simulink subsystem "Accelerometer_SubSystem"  (R2020b)
settings: Solver=VariableStepAuto  StartTime=0.0  StopTime=10.0  RelTol=1e-3
undefined symbols (not defined in the file): g, ms22g, sens, Ts, wheel
settings Model: Creator=umberto  LastModifiedBy=Musta

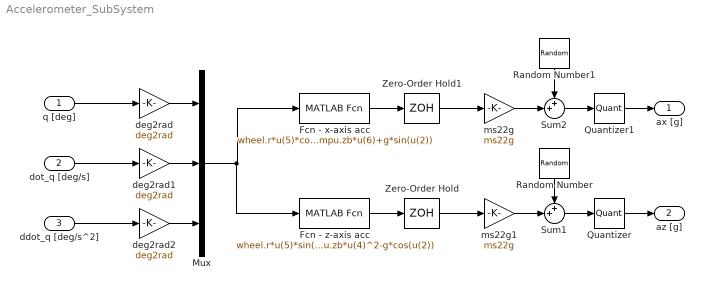
== system Accelerometer_SubSystem ==
  q [deg] : Inport
  dot_q [deg/s] : Inport  Port=2
  ddot_q [deg/s^2] : Inport  Port=3
  Fcn - x-axis acc : MATLABFcn  MATLABFcn=wheel.r*u(5)*cos(u(2))+sens.mpu.zb*u(6)+g*sin(u(2))
  Fcn - z-axis acc : MATLABFcn  MATLABFcn=wheel.r*u(5)*sin(u(2))-sens.mpu.zb*u(4)^2-g*cos(u(2))
  Mux : Mux  Inputs=3
  Quantizer : Quantizer  QuantizationInterval=sens.mpu.acc.LSB2g
  Quantizer1 : Quantizer  QuantizationInterval=sens.mpu.acc.LSB2g
  Random Number : RandomNumber  Variance=sens.mpu.acc.noisevar  SampleTime=Ts
  Random Number1 : RandomNumber  Variance=sens.mpu.acc.noisevar  SampleTime=Ts
  Sum1 : Sum  Inputs=++|
  Sum2 : Sum  Inputs=++|
  Zero-Order Hold : ZeroOrderHold  SampleTime=Ts
  Zero-Order Hold1 : ZeroOrderHold  SampleTime=Ts
  deg2rad : Gain  Gain=deg2rad
  deg2rad1 : Gain  Gain=deg2rad
  deg2rad2 : Gain  Gain=deg2rad
  ms22g : Gain  Gain=ms22g
  ms22g1 : Gain  Gain=ms22g
  ax [g] : Outport
  az [g] : Outport  Port=2
  wires:
  q [deg]/1 -> deg2rad/1
  dot_q [deg/s]/1 -> deg2rad1/1
  ddot_q [deg/s^2]/1 -> deg2rad2/1
  deg2rad1/1 -> Mux/2
  deg2rad/1 -> Mux/1
  deg2rad2/1 -> Mux/3
  Mux/1 -> Fcn - z-axis acc/1, Fcn - x-axis acc/1
  Fcn - x-axis acc/1 -> Zero-Order Hold1/1
  Fcn - z-axis acc/1 -> Zero-Order Hold/1
  Zero-Order Hold1/1 -> ms22g/1
  Zero-Order Hold/1 -> ms22g1/1
  ms22g/1 -> Sum2/2
  ms22g1/1 -> Sum1/2
  Random Number/1 -> Sum1/1
  Random Number1/1 -> Sum2/1
  Sum1/1 -> Quantizer/1
  Sum2/1 -> Quantizer1/1
  Quantizer1/1 -> ax [g]/1
  Quantizer/1 -> az [g]/1
